simulink model "sis_dinamico1_Espacio_Estados"  (R2021a)
settings: Solver=VariableStepAuto  StartTime=0.0  StopTime=50  RelTol=1e-3
values from neighbouring files (symbols this model uses):
  A = randi(3,1,3)    [Untitled2.m]    (also in Untitled5.m = 6; Untitled6.m = 6; Untitled7.m = 6; espaciosEstados.m = [-1/5,1;-1/4,-9/2])
  B = A    [Untitled2.m]    (also in Untitled5.m = 16; Untitled6.m = 16; Untitled7.m = 16; espaciosEstados.m = [0;1/4])
  C = []    [Untitled2.m]    (also in Untitled5.m = 0.383972435439; Untitled6.m = 0.383972435439; Untitled7.m = 0.383972435439; espaciosEstados.m = [1,0])
  D = A(i)    [Untitled2.m]    (also in espaciosEstados.m = [0]; operaMatrices.m = [D B(i)])
undefined symbols (not defined in the file or in its folder): denominador, numerador
settings Model: Creator=GIOVANNI  LastModifiedBy=GIOVANNI
settings SolverCC: AlgebraicLoopSolver=TrustRegion
settings DebuggingCC: SFMachineParentedDataDiag=warning

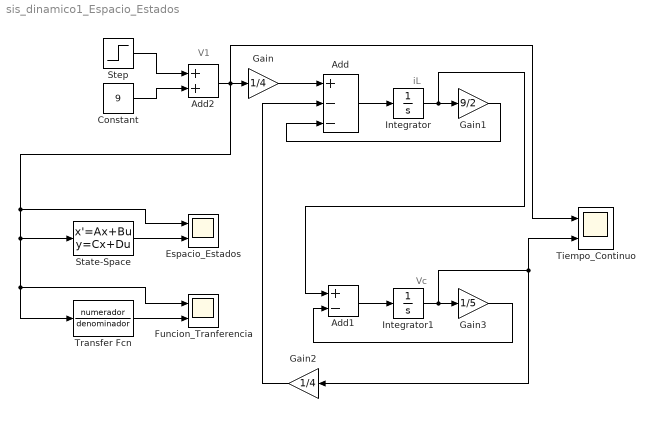
== system sis_dinamico1_Espacio_Estados ==
  note: Vc
  note: iL
  note: V1
  Add : Sum  Inputs=+--
  Add1 : Sum  Inputs=+-
  Add2 : Sum
  Constant : Constant  Value=9
  Espacio_Estados : Scope  NumInputPorts=2
  Funcion_Tranferencia : Scope  NumInputPorts=2
  Gain : Gain  Gain=1/4
  Gain1 : Gain  Gain=9/2
  Gain2 : Gain  Gain=1/4
  Gain3 : Gain  Gain=1/5
  Integrator : Integrator
  Integrator1 : Integrator
  State-Space : StateSpace  A=A  B=B  C=C  D=D  InitialCondition=0
  Step : Step  Time=5  SampleTime=0
  Tiempo_Continuo : Scope  NumInputPorts=2
  Transfer Fcn : TransferFcn  Numerator=numerador  Denominator=denominador  ParameterTunability=Optimized
  wires:
  Step/1 -> Add2/1
  Constant/1 -> Add2/2
  Add2/1 -> Espacio_Estados/1, Funcion_Tranferencia/1, Transfer Fcn/1, State-Space/1, Gain/1, Tiempo_Continuo/1
  Gain/1 -> Add/1
  Add/1 -> Integrator/1
  Integrator/1 -> Gain1/1, Add1/1
  Gain2/1 -> Add/2
  Add1/1 -> Integrator1/1
  Integrator1/1 -> Gain3/1, Gain2/1, Tiempo_Continuo/2
  Gain3/1 -> Add1/2
  Gain1/1 -> Add/3
  State-Space/1 -> Espacio_Estados/2
  Transfer Fcn/1 -> Funcion_Tranferencia/2
